simulink model "VDCHyd2022a"  (R2022a)
settings: Solver=daessc  StartTime=0.0  StopTime=simulationEndTime  FixedStep=0.001  RelTol=1e-2
values from neighbouring files (symbols this model uses):
  aux = thetaXrLB(i)    [initInertiaUpdate.m]
  Bc1_V = [0;0;0;0;0;0]    [InitializeSimulationParameters.m]
  Bc1_Vr = [0;0;0;0;0;0]    [InitializeSimulationParameters.m]
  D22Fr = [0;0;0;0;0;0]    [InitializeSimulationParameters.m]
  filtDF = init2ndOrderLowPassFilter(filtDF.cutOffFrequency,1,controller.dT)    [initializeLowPassFilters.m]
  filtDV = init2ndOrderLowPassFilter(filtDV.cutOffFrequency,1,controller.dT)    [initializeLowPassFilters.m]
  filtEnc = init2ndOrderLowPassFilter(filtEnc.cutOffFrequency,1,controller.dT)    [initializeLowPassFilters.m]
  filtPres = init2ndOrderLowPassFilter(filtPres.cutOffFrequency,1,controller.dT)    [initializeLowPassFilters.m]
  MODE = 1    [RUN_ME.m]
  s = tf('s')    [init2ndOrderLowPassFilter.m]
undefined symbols (not defined in the file or in its folder): B11_r_B11Tc1, B11_V, B11_Vr, B11Ftot_r, B12_r_B12Tc2, B12_Rot_Tc2, B12_U_Tc2, B12_V, B12_Vr, B12Ftot_r, B31_r_B31B41, B31_V, B31_Vr, B31FTot_r, B32_r_B32B42, B32_Rot_B42, B32_U_B42, B32_V, B32_Vr, B32FTot_r, B41_r_B41Tc1, B41_V, B41_Vr, B41FTot_r, B42_r_B42Tc2, B42_Rot_Tc2, B42_U_Tc2, B42_V, B42_Vr, B42FTot_r, B52_r_B52P32, B52_Rot_P32, B52_U_P32, B52_V, B52_Vr, B52Ftot_r, Bc1_r_Bc1B11, Bc1_r_Bc1B31, Bc1FTot_r, Bc2_r_Bc2B12, Bc2_r_Bc2B32, Bc2_Rot_B12, Bc2_Rot_B32, Bc2_U_B12, Bc2_U_B32, Bc2_V, Bc2_Vr, Bc2Tot_r, controller, cyl1, cyl2, cylT2, D22_V, D22_Vr, DiscIntNeverNeededParam, dq1, dq11, dq11r, dq12, dq12r ... (+119)
libraries: sm_lib x34, nesl_utility x15, simulink x11, dspinverses x1
(part 2 of 12)

== system VDCHyd2022a/sbHydraulicElements/sbHosesAndActuatorPS2 ==
  Qat2 : Inport
  Qbt2 : Inport  Port=2
  xt2 : Inport  Port=3
  dxt2 : Inport  Port=4
  sbChamberAPressure : Subsystem
  sbChamberBPressure : Subsystem
  sbLeakageFlow : Subsystem
  pat2 : Outport
  pbt2 : Outport  Port=2
  wires:
  sbChamberBPressure/1(pb) -> [pb]
  sbLeakageFlow/1(Ql) -> [Ql]
  sbChamberAPressure/1(pa) -> [pa]
  [dxp] -> sbChamberBPressure/4(dxp)
  [dxp] -> sbChamberAPressure/4(dxp)
  [xp] -> sbChamberAPressure/3(xp)
  [Qb] -> sbChamberBPressure/1(Qb)
  [xp] -> sbChamberBPressure/3(xp)
  [Ql] -> sbChamberBPressure/2(Ql)
  [Qa] -> sbChamberAPressure/1(Qa)
  [Ql] -> sbChamberAPressure/2(Ql)
  Qbt2/1 -> [Qb]  "Qbt2"
  Qat2/1 -> [Qa]  "Qat2"
  [pa] -> pat2/1  "pat2"
  [pb] -> pbt2/1  "pbt2"
  [pb] -> sbLeakageFlow/2(pb)
  [pa] -> sbLeakageFlow/1(pa)
  xt2/1 -> [xp]  "xt2"
  dxt2/1 -> [dxp]  "dxt2"

== system VDCHyd2022a/sbHydraulicElements/sbHosesAndActuatorRS1 ==
  Qa1 : Inport
  Qb1 : Inport  Port=2
  x1 : Inport  Port=3
  dx1 : Inport  Port=4
  sbChamberAPressure : Subsystem
  sbChamberBPressure : Subsystem
  sbLeakageFlow : Subsystem
  pa1 : Outport
  pb1 : Outport  Port=2
  wires:
  [dxp] -> sbChamberBPressure/4(dxp)
  [dxp] -> sbChamberAPressure/4(dxp)
  [xp] -> sbChamberAPressure/3(xp)
  [Qb] -> sbChamberBPressure/1(Qb)
  [xp] -> sbChamberBPressure/3(xp)
  [Ql] -> sbChamberBPressure/2(Ql)
  [Qa] -> sbChamberAPressure/1(Qa)
  [Ql] -> sbChamberAPressure/2(Ql)
  Qb1/1 -> [Qb]  "Qb1"
  Qa1/1 -> [Qa]  "Qa1"
  [pa] -> pa1/1  "pa1"
  [pb] -> pb1/1  "pb1"
  [pb] -> sbLeakageFlow/2(pb)
  [pa] -> sbLeakageFlow/1(pa)
  sbLeakageFlow/1(Ql) -> [Ql]
  x1/1 -> [xp]  "x1"
  dx1/1 -> [dxp]  "dx1"
  sbChamberBPressure/1(pb) -> [pb]
  sbChamberAPressure/1(pa) -> [pa]

== system VDCHyd2022a/sbHydraulicElements/sbHosesAndActuatorRS2 ==
  Qa2 : Inport
  Qb2 : Inport  Port=2
  x2 : Inport  Port=3
  dx2 : Inport  Port=4
  sbChamberAPressure : Subsystem
  sbChamberBPressure : Subsystem
  sbLeakageFlow : Subsystem
  pa2 : Outport
  pb2 : Outport  Port=2
  wires:
  dx2/1 -> [dxp]  "dx2"
  x2/1 -> [xp]  "x2"
  [pa] -> sbLeakageFlow/1(pa)
  [pb] -> sbLeakageFlow/2(pb)
  [pb] -> pb2/1  "pb2"
  [pa] -> pa2/1  "pa2"
  Qa2/1 -> [Qa]  "Qa2"
  Qb2/1 -> [Qb]  "Qb2"
  [Ql] -> sbChamberAPressure/2(Ql)
  [Qa] -> sbChamberAPressure/1(Qa)
  [Ql] -> sbChamberBPressure/2(Ql)
  [xp] -> sbChamberBPressure/3(xp)
  [Qb] -> sbChamberBPressure/1(Qb)
  [xp] -> sbChamberAPressure/3(xp)
  [dxp] -> sbChamberAPressure/4(dxp)
  [dxp] -> sbChamberBPressure/4(dxp)
  sbChamberAPressure/1(pa) -> [pa]  "pa"
  sbLeakageFlow/1(Ql) -> [Ql]  "Ql"
  sbChamberBPressure/1(pb) -> [pb]  "pb"

== system VDCHyd2022a/sbHydraulicElements/sbPistonForcePS2 ==
  note: f_{pt2} = A_{at2} p_{at2} - A_{bt2} p_{bt2}
  note: (79)
  pat2 : Inport
  pbt2 : Inport  Port=2
  Gain1 : Gain  Gain=cylT2.Aa
  Gain2 : Gain  Gain=cylT2.Ab
  Sum2 : Sum  Inputs=|+-
  fpt2 : Outport
  wires:
  Gain2/1 -> Sum2/2
  Sum2/1 -> fpt2/1  "fpt2"
  pat2/1 -> Gain1/1  "pat2"
  Gain1/1 -> Sum2/1
  pbt2/1 -> Gain2/1  "pbt2"

== system VDCHyd2022a/sbHydraulicElements/sbPistonForceRS1 ==
  note: f_{p1} = A_{a1} p_{a1} - A_{b1} p_{b1}
  note: (79)
  pa1 : Inport
  pb1 : Inport  Port=2
  Gain3 : Gain  Gain=cyl1.Aa
  Gain4 : Gain  Gain=cyl1.Ab
  Sum : Sum  Inputs=|+-
  fp1 : Outport
  wires:
  Gain3/1 -> Sum/1
  Gain4/1 -> Sum/2
  pb1/1 -> Gain4/1  "pb1"
  Sum/1 -> fp1/1  "fp1"
  pa1/1 -> Gain3/1  "pa1"

== system VDCHyd2022a/sbHydraulicElements/sbPistonForceRS2 ==
  note: (79)
  note: f_{p2} = A_{a2} p_{a2} - A_{b2} p_{b2}
  pa2 : Inport
  pb2 : Inport  Port=2
  Gain5 : Gain  Gain=cyl2.Aa
  Gain6 : Gain  Gain=cyl2.Ab
  Sum1 : Sum  Inputs=|+-
  fp2 : Outport
  wires:
  Gain6/1 -> Sum1/2
  Sum1/1 -> fp2/1  "fp2"
  Gain5/1 -> Sum1/1
  pb2/1 -> Gain6/1  "pb2"
  pa2/1 -> Gain5/1  "pa2"

== system VDCHyd2022a/sbHydraulicElements/sbPressureMeasurement ==
  pa1 : Inport
  pb1 : Inport  Port=2
  pa2 : Inport  Port=3
  pb2 : Inport  Port=4
  pat2 : Inport  Port=5
  pbt2 : Inport  Port=6
  pS : Inport  Port=7
  pR : Inport  Port=8
  Band-Limited White Noise{1..8} (8 alike) : simulink/Sources/Band-Limited White Noise  Cov=pres.measNoisePower  Ts=controller.dT  seed=[23341]
  Bus Creator1 : BusCreator  Inputs=pa1Measured,pb1Measured,pa2Measured,pb2Measured,pat2Measured,pbt2Measured,pSMeasured,pRMeasured
  Rate Transition : RateTransition  InitialCondition=initVals.pa10  OutPortSampleTime=controller.dT
  Rate Transition1 : RateTransition  InitialCondition=initVals.pb10  OutPortSampleTime=controller.dT
  Rate Transition2 : RateTransition  InitialCondition=initVals.pa20  OutPortSampleTime=controller.dT
  Rate Transition3 : RateTransition  InitialCondition=initVals.pb20  OutPortSampleTime=controller.dT
  Rate Transition4 : RateTransition  InitialCondition=initVals.pat20  OutPortSampleTime=controller.dT
  Rate Transition5 : RateTransition  InitialCondition=initVals.pbt20  OutPortSampleTime=controller.dT
  Rate Transition6 : RateTransition  InitialCondition=pres.supply  OutPortSampleTime=controller.dT
  Rate Transition7 : RateTransition  InitialCondition=pres.return  OutPortSampleTime=controller.dT
  Sum{3..10} (8 alike) : Sum  Inputs=|++
  pressuresMeasured : Outport
  wires:
  Sum4/1 -> Rate Transition1/1  "pb1Measured"
  Sum9/1 -> Rate Transition6/1  "pSMeasured"
  Sum7/1 -> Rate Transition4/1  "pat2Measured"
  Sum6/1 -> Rate Transition3/1  "pb2Measured"
  pS/1 -> Sum9/1
  Sum5/1 -> Rate Transition2/1  "pa2Measured"
  Band-Limited White Noise6/1 -> Sum3/2  "pa1MeasurementNoise"
  Band-Limited White Noise8/1 -> Sum10/2  "pRMeasurementNoise"
  pa2/1 -> Sum5/1
  Sum10/1 -> Rate Transition7/1  "pRMeasured"
  Rate Transition2/1 -> Bus Creator1/3  "pa2Measured"
  Sum8/1 -> Rate Transition5/1  "pbt2Measured"
  Rate Transition1/1 -> Bus Creator1/2  "pb1Measured"
  Rate Transition5/1 -> Bus Creator1/6  "pbt2Measured"
  pR/1 -> Sum10/1
  pat2/1 -> Sum7/1
  Rate Transition4/1 -> Bus Creator1/5  "pat2Measured"
  Rate Transition3/1 -> Bus Creator1/4  "pb2Measured"
  Rate Transition/1 -> Bus Creator1/1  "pa1Measured"
  Rate Transition7/1 -> Bus Creator1/8  "pRMeasured"
  Band-Limited White Noise2/1 -> Sum5/2  "pa2MeasurementNoise"
  Band-Limited White Noise5/1 -> Sum7/2  "pat2MeasurementNoise"
  Band-Limited White Noise3/1 -> Sum6/2  "pb2MeasurementNoise"
  Band-Limited White Noise4/1 -> Sum8/2  "pbt2MeasurementNoise"
  Sum3/1 -> Rate Transition/1  "pa1Measured"
  Band-Limited White Noise7/1 -> Sum9/2  "pSMeasurementNoise"
  Band-Limited White Noise1/1 -> Sum4/2  "pb1MeasurementNoise"
  pa1/1 -> Sum3/1
  Rate Transition6/1 -> Bus Creator1/7  "pSMeasured"
  Bus Creator1/1 -> pressuresMeasured/1  "pressuresMeasured"
  pb2/1 -> Sum6/1
  pbt2/1 -> Sum8/1
  pb1/1 -> Sum4/1

== system VDCHyd2022a/sbHydraulicElements/sbValve1SpoolDynamics ==
  note: NB! In the paper, u1v does not exist as a notion. High-bandwith valves are assumed to be used and u1v = u1. This is a fair assumption for valve like Bosch Rexroth NG6 size servo solenoid valve. Further tailoring valve dynamics per own needs could affect the flow and might require redoing control equations.
  u1 : Inport
  First Order Hold : FirstOrderHold  ErrorTolerance=inf
  rateLimiter : RateLimiter  RisingSlewLimit=valve1.riseSlewRate  FallingSlewLimit=valve1.fallSlewRate  SampleTimeMode=inherited
  saturation : Saturate  UpperLimit=valve1.uppLim  LowerLimit=valve1.lowLim
  spoolDynamics : TransferFcn  Numerator=[(valve1.nf)^2]  Denominator=[1 2*valve1.damp*(valve1.nf) (valve1.nf)^2]
  u1v : Outport
  wires:
  u1/1 -> First Order Hold/1  "u1"
  First Order Hold/1 -> saturation/1
  spoolDynamics/1 -> u1v/1  "u1v"
  rateLimiter/1 -> spoolDynamics/1
  saturation/1 -> rateLimiter/1

== system VDCHyd2022a/sbHydraulicElements/sbValve2SpoolDynamics ==
  note: NB! In the paper, u2v does not exist as a notion. High-bandwith valves are assumed to be used and u2v = u2. This is a fair assumption for valve like Bosch Rexroth NG6 size servo solenoid valve. Further tailoring valve dynamics per own needs could affect the flow and might require redoing control equations.
  u2 : Inport
  First Order Hold : FirstOrderHold  ErrorTolerance=inf
  rateLimiter : RateLimiter  RisingSlewLimit=valve2.riseSlewRate  FallingSlewLimit=valve2.fallSlewRate  SampleTimeMode=inherited
  saturation : Saturate  UpperLimit=valve2.uppLim  LowerLimit=valve2.lowLim
  spoolDynamics : TransferFcn  Numerator=[(valve2.nf)^2]  Denominator=[1 2*valve2.damp*(valve2.nf) (valve2.nf)^2]
  u2v : Outport
  wires:
  u2/1 -> First Order Hold/1  "u2"
  First Order Hold/1 -> saturation/1
  spoolDynamics/1 -> u2v/1  "u2v"
  saturation/1 -> rateLimiter/1
  rateLimiter/1 -> spoolDynamics/1

== system VDCHyd2022a/sbHydraulicElements/sbValveFlowsPS1 ==
  note: Q_{btj} = -c_{n2tj} \nu(p_{btj} - p_{r}) u_{tj} S(u_{tj}) - c_{p2tj} \nu (p_{S} - p_{btj}) u_{tj} S(-u_{tj})
  note: (83)
  note: (82)
  note: Q_{atj} = c_{p1tj} \nu(p_S - p_{atj}) u_{tj} S(u_{tj}) + c_{n1tj} \nu (p_{atj} - p_r) u_{tj} S(-u_{tj})
  pat2 : Inport
  pbt2 : Inport  Port=2
  ut2v : Inport  Port=3
  pS : Inport  Port=4
  pR : Inport  Port=5
  extensionValveFlows : MATLAB Function  TreatAsAtomicUnit=on
  Qat2 : Outport
  Qbt2 : Outport  Port=2
  wires:
  ut2v/1 -> extensionValveFlows/3(ut2v)  "ut2v"
  extensionValveFlows/1(Qat2) -> Qat2/1  "Qat2"
  pat2/1 -> extensionValveFlows/1(pat2)  "pat2"
  extensionValveFlows/2(Qbt2) -> Qbt2/1  "Qbt2"
  pR/1 -> extensionValveFlows/5(pR)  "pR"
  pS/1 -> extensionValveFlows/4(pS)  "pS"
  pbt2/1 -> extensionValveFlows/2(pbt2)  "pbt2"

== system VDCHyd2022a/sbHydraulicElements/sbValveFlowsRS1 ==
  note: (82)
  note: Q_{aj} = c_{p1j} \nu(p_S - p_{aj}) u_j S(u_j) + c_{n1j} \nu (p_{aj} - p_r) u_j S(-u_j)
  note: (83)
  note: Q_{bj} = -c_{n2j} \nu(p_{bj} - p_{r}) u_j S(u_j) - c_{p2j} \nu (p_{S} - p_{bj}) u_j S(-u_j)
  pa1 : Inport
  pb1 : Inport  Port=2
  u1v : Inport  Port=3
  pS : Inport  Port=4
  pR : Inport  Port=5
  liftValveFlows : MATLAB Function  TreatAsAtomicUnit=on
  Qa1 : Outport
  Qb1 : Outport  Port=2
  wires:
  u1v/1 -> liftValveFlows/3(u1v)  "u1v"
  pR/1 -> liftValveFlows/5(pR)  "pR"
  pb1/1 -> liftValveFlows/2(pb1)  "pb1"
  pS/1 -> liftValveFlows/4(pS)  "pS"
  liftValveFlows/1(Qa1) -> Qa1/1  "Qa1"
  liftValveFlows/2(Qb1) -> Qb1/1  "Qb1"
  pa1/1 -> liftValveFlows/1(pa1)  "pa1"

== system VDCHyd2022a/sbHydraulicElements/sbValveFlowsRS2 ==
  note: Q_{bj} = -c_{n2j} \nu(p_{bj} - p_{r}) u_j S(u_j) - c_{p2j} \nu (p_{S} - p_{bj}) u_j S(-u_j)
  note: (83)
  note: (82)
  note: Q_{aj} = c_{p1j} \nu(p_S - p_{aj}) u_j S(u_j) + c_{n1j} \nu (p_{aj} - p_r) u_j S(-u_j)
  pa2 : Inport
  pb2 : Inport  Port=2
  u2v : Inport  Port=3
  pS : Inport  Port=4
  pR : Inport  Port=5
  tiltValveFlows : MATLAB Function  TreatAsAtomicUnit=on
  Qa2 : Outport
  Qb2 : Outport  Port=2
  wires:
  u2v/1 -> tiltValveFlows/3(u2v)  "u2v"
  tiltValveFlows/1(Qa2) -> Qa2/1  "Qa2"
  pa2/1 -> tiltValveFlows/1(pa2)  "pa2"
  tiltValveFlows/2(Qb2) -> Qb2/1  "Qb2"
  pR/1 -> tiltValveFlows/5(pR)  "pR"
  pS/1 -> tiltValveFlows/4(pS)  "pS"
  pb2/1 -> tiltValveFlows/2(pb2)  "pb2"

== system VDCHyd2022a/sbHydraulicElements/sbValveT2SpoolDynamics ==
  note: NB! In the paper, ut2v does not exist as a notion. High-bandwith valves are assumed to be used and ut2v = ut2. This is a fair assumption for valve like Bosch Rexroth NG6 size servo solenoid valve. Further tailoring valve dynamics per own needs could affect the flow and might require redoing control equations.
  ut2 : Inport
  First Order Hold : FirstOrderHold  ErrorTolerance=inf
  rateLimiter : RateLimiter  RisingSlewLimit=valveT2.riseSlewRate  FallingSlewLimit=valveT2.fallSlewRate  SampleTimeMode=inherited
  saturation : Saturate  UpperLimit=valveT2.uppLim  LowerLimit=valveT2.lowLim
  spoolDynamics : TransferFcn  Numerator=[(valveT2.nf)^2]  Denominator=[1 2*valveT2.damp*(valveT2.nf) (valveT2.nf)^2]
  ut2v : Outport
  wires:
  ut2/1 -> First Order Hold/1  "ut2"
  First Order Hold/1 -> saturation/1
  spoolDynamics/1 -> ut2v/1  "ut2v"
  saturation/1 -> rateLimiter/1
  rateLimiter/1 -> spoolDynamics/1

== system VDCHyd2022a/sbHydraulicManipulatorSimscape/sbBase ==
  note: Defines world (W) frame.
  note: Resembles an ideal encoder.
  BaseR_To_W : sm_lib/Frames and Transforms/Rigid Transform  TranslationMethod=None  TranslationStandardOffset=0  TranslationLengthUnit=m  TranslationStandardAxis=+Z  TranslationCartesianOffset=[0 0 0]  TranslationROffset=0  TranslationROffsetUnits=m  TranslationZOffset=0  TranslationZOffsetUnits=m  TranslationThetaOffset=0  TranslationThetaOffsetUnits=deg  RotationMethod=StandardAxis  RotationAngleUnits=deg  RotationStandardAxis=+Y  RotationAngle=90  RotationArbitraryAxis=[0 0 1]  FollAlignAxisA=+X  BaseAlignAxisA=+Y  FollAlignAxisB=+Y  BaseAlignAxisB=+Z  RotationSequenceAxes=FollowerAxes  RotationSequence=XYX  RotationSequenceAngles=[0 0 0]  RotationSequenceAnglesUnits=deg  RotationMatrix=[1 0 0; 0 1 0; 0 0 1]
  BaseSolid : sm_lib/Body Elements/File Solid  ExtGeomFileName=01_BaseGP.STEP  UnitType=FromFile  ExtGeomFileUnits=m  StepReaderType=OCC  ExportConvexHullGeometry=off  InertiaType=Custom  Mass=307.29601379  MassUnits=kg  CenterOfMass=[0 -0.01488967 0.02139206]  CenterOfMassUnits=m  MomentsOfInertia=[29.78955950 5.25917100 29.30269608]  MomentsOfInertiaUnits=kg*m^2  ProductsOfInertia=[-3.89461427 -0.00003008 -0.00000910]  ProductsOfInertiaUnits=kg*m^2  BasedOnType=Density  Density=7300  DensityUnits=kg/m^3  DoExposeReferenceFrame=on  SerializedFrames=<Frames><Frame><Id>Frame1</Id><Value><Name>F2</Name><Origin><Source>GeometricFeature</Source><FeatureName>cylindrical surface 2</FeatureName></Origin><PrimaryAxis><DefinedDirection>+X</DefinedDirection><Source>ReferenceFrame</Source><SourceDirection>-Z</SourceDirection><FeatureName></FeatureName></PrimaryAxis><SecondaryAxis><DefinedDirection>+Y</DefinedDirection><Source>ReferenceFrame</Source><SourceDirection>+Y</SourceDirection><FeatureName></FeatureName></SecondaryAxis></Value></Frame><Frame><Id>Frame2</Id><Value><Name>F1</Name><Origin><Source>GeometricFeature</Source><FeatureName>cylindrical surface 1</FeatureName></Origin><PrimaryAxis><DefinedDirection>-X</DefinedDirection><Source>ReferenceFrame</Source><SourceDirection>+Z</SourceDirection><FeatureName></FeatureName></PrimaryAxis><SecondaryAxis><DefinedDirection>+Y</DefinedDirection><Source>ReferenceFrame</Source><SourceDirection>+Y</SourceDirection><FeatureName></FeatureName></SecondaryAxis></Value></Frame><Frame><Id>Frame3</Id><Value><Name>Bc1</Name><Origin><Source>GeometricFeature</Source><FeatureName>cylindrical surface 1</FeatureName></Origin><PrimaryAxis><DefinedDirection>+X</DefinedDirection><Source>GeometricFeature</Source><SourceDirection>+Z</SourceDirection><FeatureName>segment 135</FeatureName></PrimaryAxis><SecondaryAxis><DefinedDirection>+Y</DefinedDirection><Source>ReferenceFrame</Source><SourceDirection>+Z</SourceDirection><FeatureName></FeatureName></SecondaryAxis></Value></Frame></Frames>  GraphicType=FromGeometry  MarkerShape=Sphere  MarkerSize=10  GraphicVisPropType=SimpleVisualProperties  GraphicDiffuseColor=[134 134 71]/255  GraphicSpecularColor=[0.5 0.5 0.5 1.0]  GraphicAmbientColor=[0.15 0.15 0.15 1.0]  GraphicEmissiveColor=[0.0 0.0 0.0 1.0]  GraphicShininess=75  GraphicOpacity=1.0
  PS-Simulink Converter : nesl_utility/PS-Simulink Converter  PhysicalDomain=network_engine_domain  SubClassName=ps_output  LeftPortType=input  RightPortType=output  PseudoPeriodic=off  Frequencies=[]  VectorFormat=inherit  Unit=inherit  AffineConversion=off
      settings: SourceProductBaseCode=SS,PW,VE
  theta1Rotation : sm_lib/Joints/Revolute Joint  JointMode=Normal  SenseConstraintForce=off  SenseConstraintForceX=off  SenseConstraintForceY=off  SenseConstraintForceZ=off  SenseConstraintTorque=off  SenseConstraintTorqueX=off  SenseConstraintTorqueY=off  SenseConstraintTorqueZ=off  SenseTotalForce=off  SenseTotalForceX=off  SenseTotalForceY=off  SenseTotalForceZ=off  SenseTotalTorque=off  SenseTotalTorqueX=off  SenseTotalTorqueY=off  SenseTotalTorqueZ=off  CompositeWrenchDir=FollowerOnBase  CompositeWrenchFrame=BaseFrame  EquilibriumPosition=0  EquilibriumPositionUnits=rad  SpringStiffness=0  SpringStiffnessUnits=N*m/rad  DampingCoefficient=revJoint1.damp  DampingCoefficientUnits=N*m/(rad/s)  TorqueActuationMode=NoTorque  MotionActuationMode=ComputedMotion  SensePosition=on  SenseVelocity=off  SenseAcceleration=off  SenseTorqueForce=off  SenseLowerLimitTorqueForce=off  SenseUpperLimitTorqueForce=off  LowerLimitSpecify=off  LowerLimitBound=-90  LowerLimitBoundUnits=deg  LowerLimitStiffness=1e4  LowerLimitStiffnessUnits=N*m/deg  LowerLimitDamping=10  LowerLimitDampingUnits=N*m/(deg/s)  LowerLimitTransitionRegionWidth=0.1  LowerLimitTransitionRegionWidthUnits=deg  UpperLimitSpecify=off  UpperLimitBound=90  UpperLimitBoundUnits=deg  UpperLimitStiffness=1e4  UpperLimitStiffnessUnits=N*m/deg  UpperLimitDamping=10  UpperLimitDampingUnits=N*m/(deg/s)  UpperLimitTransitionRegionWidth=0.1  UpperLimitTransitionRegionWidthUnits=deg  PositionTargetSpecify=on  PositionTargetPriority=High  PositionTargetValue=initVals.theta10  PositionTargetValueUnits=rad  VelocityTargetSpecify=on  VelocityTargetPriority=High  VelocityTargetValue=0  VelocityTargetValueUnits=rad/s
  W : PMIOPort  Side=Left
  Bc1 : PMIOPort  Port=2  Side=Left
  F1 : PMIOPort  Port=3  Side=Right
  F2_rot : PMIOPort  Port=4  Side=Right
  theta1 : Outport
  wires:
  PS-Simulink Converter/1 -> theta1/1
  connections:
  BaseR_To_W/LConn1 -- BaseSolid/RConn1
  W/RConn1 -- BaseR_To_W/RConn1
  theta1Rotation/LConn1 -- BaseSolid/LConn1
  F2_rot/RConn1 -- theta1Rotation/RConn1
  F1/RConn1 -- BaseSolid/LConn2
  Bc1/RConn1 -- BaseSolid/RConn2
  PS-Simulink Converter/LConn1 -- theta1Rotation/RConn2

== system VDCHyd2022a/sbHydraulicManipulatorSimscape/sbEndMassObject ==
  EndObjectMass : sm_lib/Body Elements/File Solid  ExtGeomFileName=10_ObjectGP.STEP  UnitType=FromFile  ExtGeomFileUnits=m  StepReaderType=OCC  ExportConvexHullGeometry=off  InertiaType=Custom  Mass=570.18877059  MassUnits=kg  CenterOfMass=[2.16142487 0.01347152 0.06601658]  CenterOfMassUnits=m  MomentsOfInertia=[46.81220713 72.19317437 67.11012925]  MomentsOfInertiaUnits=kg*m^2  ProductsOfInertia=[0.04641137 0.08825278 0.37588204]  ProductsOfInertiaUnits=kg*m^2  BasedOnType=Density  Density=7850  DensityUnits=kg/m^3  DoExposeReferenceFrame=off  SerializedFrames=<Frames><Frame><Id>Frame1</Id><Value><Name>P32p</Name><Origin><Source>GeometricFeature</Source><FeatureName>circular curve 7</FeatureName></Origin><PrimaryAxis><DefinedDirection>+Y</DefinedDirection><Source>GeometricFeature</Source><SourceDirection>+Z</SourceDirection><FeatureName>segment 159</FeatureName></PrimaryAxis><SecondaryAxis><DefinedDirection>+X</DefinedDirection><Source>ReferenceFrame</Source><SourceDirection>+X</SourceDirection><FeatureName></FeatureName></SecondaryAxis></Value></Frame><Frame><Id>Frame2</Id><Value><Name>D22</Name><Origin><Source>GeometricFeature</Source><FeatureName>planar surface 154</FeatureName></Origin><PrimaryAxis><DefinedDirection>+Z</DefinedDirection><Source>ReferenceFrame</Source><SourceDirection>+Z</SourceDirection><FeatureName></FeatureName></PrimaryAxis><SecondaryAxis><DefinedDirection>+X</DefinedDirection><Source>ReferenceFrame</Source><SourceDirection>+X</SourceDirection><FeatureName></FeatureName></SecondaryAxis></Value></Frame></Frames>  GraphicType=FromGeometry  MarkerShape=Sphere  MarkerSize=10  GraphicVisPropType=SimpleVisualProperties  GraphicDiffuseColor=[255 9 134]/255  GraphicSpecularColor=[0.5 0.5 0.5 1.0]  GraphicAmbientColor=[0.15 0.15 0.15 1.0]  GraphicEmissiveColor=[0.0 0.0 0.0 1.0]  GraphicShininess=75  GraphicOpacity=1.0
  P32p_to_P32 : sm_lib/Frames and Transforms/Rigid Transform  TranslationMethod=StandardAxis  TranslationStandardOffset=17  TranslationLengthUnit=mm  TranslationStandardAxis=+Z  TranslationCartesianOffset=[0 0 0]  TranslationROffset=0  TranslationROffsetUnits=m  TranslationZOffset=0  TranslationZOffsetUnits=m  TranslationThetaOffset=0  TranslationThetaOffsetUnits=deg  RotationMethod=None  RotationAngleUnits=deg  RotationStandardAxis=+Y  RotationAngle=-90  RotationArbitraryAxis=[0 0 1]  FollAlignAxisA=+X  BaseAlignAxisA=+Y  FollAlignAxisB=+Y  BaseAlignAxisB=+Z  RotationSequenceAxes=FollowerAxes  RotationSequence=XYX  RotationSequenceAngles=[0 0 0]  RotationSequenceAnglesUnits=deg  RotationMatrix=[1 0 0; 0 1 0; 0 0 1]
  P32 : PMIOPort  Side=Left
  D22 : PMIOPort  Port=2  Side=Left
  connections:
  EndObjectMass/LConn1 -- P32p_to_P32/LConn1
  P32p_to_P32/RConn1 -- P32/RConn1
  D22/RConn1 -- EndObjectMass/RConn1

== system VDCHyd2022a/sbHydraulicManipulatorSimscape/sbLiftCylinderAndLiftPiston ==
  note: Friction force...
  fp1 : Inport
  B31p_to_B31pAux : sm_lib/Frames and Transforms/Rigid Transform  TranslationMethod=None  TranslationStandardOffset=0  TranslationLengthUnit=m  TranslationStandardAxis=+Z  TranslationCartesianOffset=[0 0 0]  TranslationROffset=0  TranslationROffsetUnits=m  TranslationZOffset=0  TranslationZOffsetUnits=m  TranslationThetaOffset=0  TranslationThetaOffsetUnits=deg  RotationMethod=StandardAxis  RotationAngleUnits=deg  RotationStandardAxis=+Y  RotationAngle=90  RotationArbitraryAxis=[0 0 1]  FollAlignAxisA=+X  BaseAlignAxisA=+Y  FollAlignAxisB=+Y  BaseAlignAxisB=+Z  RotationSequenceAxes=FollowerAxes  RotationSequence=XYX  RotationSequenceAngles=[0 0 0]  RotationSequenceAnglesUnits=deg  RotationMatrix=[1 0 0; 0 1 0; 0 0 1]
  B41Aux_to_B41 : sm_lib/Frames and Transforms/Rigid Transform  TranslationMethod=None  TranslationStandardOffset=0  TranslationLengthUnit=m  TranslationStandardAxis=+Z  TranslationCartesianOffset=[0 0 0]  TranslationROffset=0  TranslationROffsetUnits=m  TranslationZOffset=0  TranslationZOffsetUnits=m  TranslationThetaOffset=0  TranslationThetaOffsetUnits=deg  RotationMethod=StandardAxis  RotationAngleUnits=deg  RotationStandardAxis=+Y  RotationAngle=-90  RotationArbitraryAxis=[0 0 1]  FollAlignAxisA=+X  BaseAlignAxisA=+Y  FollAlignAxisB=+Y  BaseAlignAxisB=+Z  RotationSequenceAxes=FollowerAxes  RotationSequence=XYX  RotationSequenceAngles=[0 0 0]  RotationSequenceAnglesUnits=deg  RotationMatrix=[1 0 0; 0 1 0; 0 0 1]
  Constant : Constant  Value=settings.actuatorFrictionON
  Constant1 : Constant  Value=0
  LiftCylinderSolid : sm_lib/Body Elements/File Solid  ExtGeomFileName=03_LiftCylGP.STEP  UnitType=FromFile  ExtGeomFileUnits=m  StepReaderType=OCC  ExportConvexHullGeometry=off  InertiaType=Custom  Mass=17.36281648  MassUnits=kg  CenterOfMass=[0 0.31781210 0]  CenterOfMassUnits=m  MomentsOfInertia=[0.90735702 0.03150902 0.90763033]  MomentsOfInertiaUnits=kg*m^2  ProductsOfInertia=[0 0 0]  ProductsOfInertiaUnits=kg*m^2  BasedOnType=Density  Density=7300  DensityUnits=kg/m^3  DoExposeReferenceFrame=off  SerializedFrames=<Frames><Frame><Id>Frame1</Id><Value><Name>B31</Name><Origin><Source>GeometricFeature</Source><FeatureName>cylindrical surface 11</FeatureName></Origin><PrimaryAxis><DefinedDirection>+X</DefinedDirection><Source>ReferenceFrame</Source><SourceDirection>+Y</SourceDirection><FeatureName></FeatureName></PrimaryAxis><SecondaryAxis><DefinedDirection>+Y</DefinedDirection><Source>ReferenceFrame</Source><SourceDirection>-X</SourceDirection><FeatureName></FeatureName></SecondaryAxis></Value></Frame><Frame><Id>Frame2</Id><Value><Name>B31p</Name><Origin><Source>GeometricFeature</Source><FeatureName>planar surface 4</FeatureName></Origin><PrimaryAxis><DefinedDirection>+X</DefinedDirection><Source>ReferenceFrame</Source><SourceDirection>+Y</SourceDirection><FeatureName></FeatureName></PrimaryAxis><SecondaryAxis><DefinedDirection>+Y</DefinedDirection><Source>ReferenceFrame</Source><SourceDirection>-X</SourceDirection><FeatureName></FeatureName></SecondaryAxis></Value></Frame></Frames>  GraphicType=FromGeometry  MarkerShape=Sphere  MarkerSize=10  GraphicVisPropType=SimpleVisualProperties  GraphicDiffuseColor=[1 1 119]/255  GraphicSpecularColor=[0.5 0.5 0.5 1.0]  GraphicAmbientColor=[0.15 0.15 0.15 1.0]  GraphicEmissiveColor=[0.0 0.0 0.0 1.0]  GraphicShininess=75  GraphicOpacity=1.0
  LiftPistonSolid : sm_lib/Body Elements/File Solid  ExtGeomFileName=04_LiftPistGP.STEP  UnitType=FromFile  ExtGeomFileUnits=m  StepReaderType=OCC  ExportConvexHullGeometry=off  InertiaType=Custom  Mass=10.34519231  MassUnits=kg  CenterOfMass=[0 0.32981882 0]  CenterOfMassUnits=m  MomentsOfInertia=[0.55759812 0.00370720 0.55785997]  MomentsOfInertiaUnits=kg*m^2  ProductsOfInertia=[0 0 0]  ProductsOfInertiaUnits=kg*m^2  BasedOnType=Density  Density=7800  DensityUnits=kg/m^3  DoExposeReferenceFrame=off  SerializedFrames=<Frames><Frame><Id>Frame2</Id><Value><Name>B41</Name><Origin><Source>GeometricFeature</Source><FeatureName>planar surface 2</FeatureName></Origin><PrimaryAxis><DefinedDirection>+X</DefinedDirection><Source>ReferenceFrame</Source><SourceDirection>+Y</SourceDirection><FeatureName></FeatureName></PrimaryAxis><SecondaryAxis><DefinedDirection>+Y</DefinedDirection><Source>ReferenceFrame</Source><SourceDirection>-X</SourceDirection><FeatureName></FeatureName></SecondaryAxis></Value></Frame><Frame><Id>Frame3</Id><Value><Name>P11</Name><Origin><Source>GeometricFeature</Source><FeatureName>cylindrical surface 8</FeatureName></Origin><PrimaryAxis><DefinedDirection>+X</DefinedDirection><Source>ReferenceFrame</Source><SourceDirection>+Y</SourceDirection><FeatureName></FeatureName></PrimaryAxis><SecondaryAxis><DefinedDirection>+Y</DefinedDirection><Source>ReferenceFrame</Source><SourceDirection>-X</SourceDirection><FeatureName></FeatureName></SecondaryAxis></Value></Frame></Frames>  GraphicType=FromGeometry  MarkerShape=Sphere  MarkerSize=10  GraphicVisPropType=SimpleVisualProperties  GraphicDiffuseColor=[9 232 232]/255  GraphicSpecularColor=[0.5 0.5 0.5 1.0]  GraphicAmbientColor=[0.15 0.15 0.15 1.0]  GraphicEmissiveColor=[0.0 0.0 0.0 1.0]  GraphicShininess=75  GraphicOpacity=1.0
  PS-Sim1 : nesl_utility/PS-Simulink Converter  PhysicalDomain=network_engine_domain  SubClassName=ps_output  LeftPortType=input  RightPortType=output  PseudoPeriodic=off  Frequencies=[]  VectorFormat=1-D array  Unit=inherit  AffineConversion=off
      settings: SourceProductBaseCode=SS,PW,VE
  PS-Sim2 : nesl_utility/PS-Simulink Converter  PhysicalDomain=network_engine_domain  SubClassName=ps_output  LeftPortType=input  RightPortType=output  PseudoPeriodic=off  Frequencies=[]  VectorFormat=1-D array  Unit=inherit  AffineConversion=off
      settings: SourceProductBaseCode=SS,PW,VE
  Simulink-PS Converter : nesl_utility/Simulink-PS Converter  PhysicalDomain=network_engine_domain  SubClassName=ps_input  LeftPortType=input  RightPortType=output  PseudoPeriodic=off  Frequencies=[]  NoiseDistribution=none  NoiseParameters=[]  Unit=1  AffineConversion=off  FilteringAndDerivatives=provide  SimscapeFilterOrder=1  InputFilterTimeConstant=0.001  UdotUserProvided=0
      settings: SourceProductBaseCode=SS,PW,VE
  Sum : Sum  Inputs=|+-
  Switch : Switch  Criteria=u2 > Threshold  SaturateOnIntegerOverflow=off  InputSameDT=off
  q11Rotation : sm_lib/Joints/Revolute Joint  JointMode=Normal  SenseConstraintForce=off  SenseConstraintForceX=off  SenseConstraintForceY=off  SenseConstraintForceZ=off  SenseConstraintTorque=off  SenseConstraintTorqueX=off  SenseConstraintTorqueY=off  SenseConstraintTorqueZ=off  SenseTotalForce=off  SenseTotalForceX=off  SenseTotalForceY=off  SenseTotalForceZ=off  SenseTotalTorque=off  SenseTotalTorqueX=off  SenseTotalTorqueY=off  SenseTotalTorqueZ=off  CompositeWrenchDir=FollowerOnBase  CompositeWrenchFrame=BaseFrame  EquilibriumPosition=0  EquilibriumPositionUnits=rad  SpringStiffness=0  SpringStiffnessUnits=N*m/rad  DampingCoefficient=revJoint1.damp  DampingCoefficientUnits=N*m/(rad/s)  TorqueActuationMode=NoTorque  MotionActuationMode=ComputedMotion  SensePosition=off  SenseVelocity=off  SenseAcceleration=off  SenseTorqueForce=off  SenseLowerLimitTorqueForce=off  SenseUpperLimitTorqueForce=off  LowerLimitSpecify=off  LowerLimitBound=-90  LowerLimitBoundUnits=deg  LowerLimitStiffness=1e4  LowerLimitStiffnessUnits=N*m/deg  LowerLimitDamping=10  LowerLimitDampingUnits=N*m/(deg/s)  LowerLimitTransitionRegionWidth=0.1  LowerLimitTransitionRegionWidthUnits=deg  UpperLimitSpecify=off  UpperLimitBound=90  UpperLimitBoundUnits=deg  UpperLimitStiffness=1e4  UpperLimitStiffnessUnits=N*m/deg  UpperLimitDamping=10  UpperLimitDampingUnits=N*m/(deg/s)  UpperLimitTransitionRegionWidth=0.1  UpperLimitTransitionRegionWidthUnits=deg  PositionTargetSpecify=off  PositionTargetPriority=High  PositionTargetValue=0  PositionTargetValueUnits=deg  VelocityTargetSpecify=off  VelocityTargetPriority=High  VelocityTargetValue=0  VelocityTargetValueUnits=deg/s
  q12Rotation : sm_lib/Joints/Revolute Joint  JointMode=Normal  SenseConstraintForce=off  SenseConstraintForceX=off  SenseConstraintForceY=off  SenseConstraintForceZ=off  SenseConstraintTorque=off  SenseConstraintTorqueX=off  SenseConstraintTorqueY=off  SenseConstraintTorqueZ=off  SenseTotalForce=off  SenseTotalForceX=off  SenseTotalForceY=off  SenseTotalForceZ=off  SenseTotalTorque=off  SenseTotalTorqueX=off  SenseTotalTorqueY=off  SenseTotalTorqueZ=off  CompositeWrenchDir=FollowerOnBase  CompositeWrenchFrame=BaseFrame  EquilibriumPosition=0  EquilibriumPositionUnits=rad  SpringStiffness=0  SpringStiffnessUnits=N*m/rad  DampingCoefficient=revJoint1.damp  DampingCoefficientUnits=N*m/(rad/s)  TorqueActuationMode=NoTorque  MotionActuationMode=ComputedMotion  SensePosition=off  SenseVelocity=off  SenseAcceleration=off  SenseTorqueForce=off  SenseLowerLimitTorqueForce=off  SenseUpperLimitTorqueForce=off  LowerLimitSpecify=off  LowerLimitBound=-90  LowerLimitBoundUnits=deg  LowerLimitStiffness=1e4  LowerLimitStiffnessUnits=N*m/deg  LowerLimitDamping=10  LowerLimitDampingUnits=N*m/(deg/s)  LowerLimitTransitionRegionWidth=0.1  LowerLimitTransitionRegionWidthUnits=deg  UpperLimitSpecify=off  UpperLimitBound=90  UpperLimitBoundUnits=deg  UpperLimitStiffness=1e4  UpperLimitStiffnessUnits=N*m/deg  UpperLimitDamping=10  UpperLimitDampingUnits=N*m/(deg/s)  UpperLimitTransitionRegionWidth=0.1  UpperLimitTransitionRegionWidthUnits=deg  PositionTargetSpecify=off  PositionTargetPriority=High  PositionTargetValue=0  PositionTargetValueUnits=deg  VelocityTargetSpecify=off  VelocityTargetPriority=High  VelocityTargetValue=0  VelocityTargetValueUnits=deg/s
  sbFrictionForceRS1 : Subsystem
  x1-translation : sm_lib/Joints/Prismatic Joint  JointMode=Normal  SenseConstraintForce=off  SenseConstraintForceX=off  SenseConstraintForceY=off  SenseConstraintForceZ=off  SenseConstraintTorque=off  SenseConstraintTorqueX=off  SenseConstraintTorqueY=off  SenseConstraintTorqueZ=off  SenseTotalForce=off  SenseTotalForceX=off  SenseTotalForceY=off  SenseTotalForceZ=off  SenseTotalTorque=off  SenseTotalTorqueX=off  SenseTotalTorqueY=off  SenseTotalTorqueZ=off  CompositeWrenchDir=FollowerOnBase  CompositeWrenchFrame=FollowerFrame  EquilibriumPosition=0  EquilibriumPositionUnits=m  SpringStiffness=0  SpringStiffnessUnits=N/m  DampingCoefficient=0  DampingCoefficientUnits=N/(m/s)  TorqueActuationMode=InputTorque  MotionActuationMode=ComputedMotion  SensePosition=on  SenseVelocity=on  SenseAcceleration=off  SenseTorqueForce=off  SenseLowerLimitTorqueForce=off  SenseUpperLimitTorqueForce=off  LowerLimitSpecify=on  LowerLimitBound=0  LowerLimitBoundUnits=m  LowerLimitStiffness=1e6  LowerLimitStiffnessUnits=N/m  LowerLimitDamping=1e3  LowerLimitDampingUnits=N/(m/s)  LowerLimitTransitionRegionWidth=1e-4  LowerLimitTransitionRegionWidthUnits=m  UpperLimitSpecify=on  UpperLimitBound=cyl1.sp  UpperLimitBoundUnits=m  UpperLimitStiffness=1e6  UpperLimitStiffnessUnits=N/m  UpperLimitDamping=1e3  UpperLimitDampingUnits=N/(m/s)  UpperLimitTransitionRegionWidth=1e-4  UpperLimitTransitionRegionWidthUnits=m  PositionTargetSpecify=on  PositionTargetPriority=Low  PositionTargetValue=0.4  PositionTargetValueUnits=m  VelocityTargetSpecify=on  VelocityTargetPriority=High  VelocityTargetValue=0  VelocityTargetValueUnits=m/s
  B31 : PMIOPort  Side=Left
  B41 : PMIOPort  Port=2  Side=Left
  F1 : PMIOPort  Port=3  Side=Right
  F3 : PMIOPort  Port=4  Side=Right
  x1 : Outport
  dx1 : Outport  Port=2
  wires:
  PS-Sim1/1 -> x1/1
  fp1/1 -> sbFrictionForceRS1/2(fp1), Sum/1
  Sum/1 -> Simulink-PS Converter/1
  Switch/1 -> Sum/2
  PS-Sim2/1 -> sbFrictionForceRS1/1(dx1), dx1/1
  Constant1/1 -> Switch/3
  sbFrictionForceRS1/1(ff1) -> Switch/1
  Constant/1 -> Switch/2
  connections:
  B31p_to_B31pAux/LConn1 -- LiftCylinderSolid/RConn1
  x1-translation/RConn1 -- B41Aux_to_B41/LConn1
  q11Rotation/RConn1 -- B31/RConn1 -- LiftCylinderSolid/LConn1
  LiftPistonSolid/LConn1 -- B41/RConn1 -- B41Aux_to_B41/RConn1
  B31p_to_B31pAux/RConn1 -- x1-translation/LConn1
  q11Rotation/LConn1 -- F1/RConn1
  q12Rotation/LConn1 -- LiftPistonSolid/RConn1
  q12Rotation/RConn1 -- F3/RConn1
  PS-Sim1/LConn1 -- x1-translation/RConn2
  Simulink-PS Converter/RConn1 -- x1-translation/LConn2
  x1-translation/RConn3 -- PS-Sim2/LConn1

== system VDCHyd2022a/sbHydraulicManipulatorSimscape/sbLiftLink ==
  note: Resembles an ideal encoder.
  LiftLinkSolid : sm_lib/Body Elements/File Solid  ExtGeomFileName=02_LiftLinkGP.STEP  UnitType=FromFile  ExtGeomFileUnits=m  StepReaderType=OCC  ExportConvexHullGeometry=off  InertiaType=Custom  Mass=80.11363010  MassUnits=kg  CenterOfMass=[0 -0.04248930 0.76135480]  CenterOfMassUnits=m  MomentsOfInertia=[16.37344274 16.11821222 0.72023904]  MomentsOfInertiaUnits=kg*m^2  ProductsOfInertia=[-0.55980815 0 0]  ProductsOfInertiaUnits=kg*m^2  BasedOnType=Mass  Density=7300  DensityUnits=kg/m^3  DoExposeReferenceFrame=off  SerializedFrames=<Frames><Frame><Id>Frame1</Id><Value><Name>F5</Name><Origin><Source>GeometricFeature</Source><FeatureName>cylindrical surface 18</FeatureName></Origin><PrimaryAxis><DefinedDirection>+X</DefinedDirection><Source>ReferenceFrame</Source><SourceDirection>+Z</SourceDirection><FeatureName></FeatureName></PrimaryAxis><SecondaryAxis><DefinedDirection>+Y</DefinedDirection><Source>ReferenceFrame</Source><SourceDirection>+Y</SourceDirection><FeatureName></FeatureName></SecondaryAxis></Value></Frame><Frame><Id>Frame2</Id><Value><Name>F2rot</Name><Origin><Source>GeometricFeature</Source><FeatureName>cylindrical surface 7</FeatureName></Origin><PrimaryAxis><DefinedDirection>+X</DefinedDirection><Source>ReferenceFrame</Source><SourceDirection>+Z</SourceDirection><FeatureName></FeatureName></PrimaryAxis><SecondaryAxis><DefinedDirection>+Y</DefinedDirection><Source>ReferenceFrame</Source><SourceDirection>+Y</SourceDirection><FeatureName></FeatureName></SecondaryAxis></Value></Frame><Frame><Id>Frame3</Id><Value><Name>F3</Name><Origin><Source>GeometricFeature</Source><FeatureName>cylindrical surface 8</FeatureName></Origin><PrimaryAxis><DefinedDirection>+X</DefinedDirection><Source>ReferenceFrame</Source><SourceDirection>+Z</SourceDirection><FeatureName></FeatureName></PrimaryAxis><SecondaryAxis><DefinedDirection>+Y</DefinedDirection><Source>ReferenceFrame</Source><SourceDirection>+Y</SourceDirection><FeatureName></FeatureName></SecondaryAxis></Value></Frame><Frame><Id>Frame4</Id><Value><Name>F4</Name><Origin><Source>GeometricFeature</Source><FeatureName>cylindrical surface 9</FeatureName></Origin><PrimaryAxis><DefinedDirection>+X</DefinedDirection><Source>ReferenceFrame</Source><SourceDirection>+Z</SourceDirection><FeatureName></FeatureName></PrimaryAxis><SecondaryAxis><DefinedDirection>+Y</DefinedDirection><Source>ReferenceFrame</Source><SourceDirection>+Y</SourceDirection><FeatureName></FeatureName></SecondaryAxis></Value></Frame><Frame><Id>Frame5</Id><Value><Name>B11</Name><Origin><Source>GeometricFeature</Source><FeatureName>cylindrical surface 7</FeatureName></Origin><PrimaryAxis><DefinedDirection>+X</DefinedDirection><Source>GeometricFeature</Source><SourceDirection>+Z</SourceDirection><FeatureName>segment 149</FeatureName></PrimaryAxis><SecondaryAxis><DefinedDirection>+Y</DefinedDirection><Source>ReferenceFrame</Source><SourceDirection>+Y</SourceDirection><FeatureName></FeatureName></SecondaryAxis></Value></Frame><Frame><Id>Frame6</Id><Value><Name>Bc2</Name><Origin><Source>GeometricFeature</Source><FeatureName>cylindrical surface 9</FeatureName></Origin><PrimaryAxis><DefinedDirection>+X</DefinedDirection><Source>GeometricFeature</Source><SourceDirection>+Z</SourceDirection><FeatureName>segment 153</FeatureName></PrimaryAxis><SecondaryAxis><DefinedDirection>+Y</DefinedDirection><Source>ReferenceFrame</Source><SourceDirection>+Y</SourceDirection><FeatureName></FeatureName></SecondaryAxis></Value></Frame><Frame><Id>Frame7</Id><Value><Name>Tc1</Name><Origin><Source>GeometricFeature</Source><FeatureName>cylindrical surface 8</FeatureName></Origin><PrimaryAxis><DefinedDirection>+X</DefinedDirection><Source>GeometricFeature</Source><SourceDirection>+Z</SourceDirection><FeatureName>segment 149</FeatureName></PrimaryAxis><SecondaryAxis><DefinedDirection>+Y</DefinedDirection><Source>ReferenceFrame</Source><SourceDirection>+Y</SourceDirection><FeatureName></FeatureName></SecondaryAxis></Value></Frame></Frames>  GraphicType=FromGeometry  MarkerShape=Sphere  MarkerSize=10  GraphicVisPropType=SimpleVisualProperties  GraphicDiffuseColor=[255 192 138]/255  GraphicSpecularColor=[0.5 0.5 0.5 1.0]  GraphicAmbientColor=[0.15 0.15 0.15 1.0]  GraphicEmissiveColor=[0.0 0.0 0.0 1.0]  GraphicShininess=75  GraphicOpacity=1.0
  PS-Simulink Converter : nesl_utility/PS-Simulink Converter  PhysicalDomain=network_engine_domain  SubClassName=ps_output  LeftPortType=input  RightPortType=output  PseudoPeriodic=off  Frequencies=[]  VectorFormat=inherit  Unit=inherit  AffineConversion=off
      settings: SourceProductBaseCode=SS,PW,VE
  theta2Rotation : sm_lib/Joints/Revolute Joint  JointMode=Normal  SenseConstraintForce=off  SenseConstraintForceX=off  SenseConstraintForceY=off  SenseConstraintForceZ=off  SenseConstraintTorque=off  SenseConstraintTorqueX=off  SenseConstraintTorqueY=off  SenseConstraintTorqueZ=off  SenseTotalForce=off  SenseTotalForceX=off  SenseTotalForceY=off  SenseTotalForceZ=off  SenseTotalTorque=off  SenseTotalTorqueX=off  SenseTotalTorqueY=off  SenseTotalTorqueZ=off  CompositeWrenchDir=FollowerOnBase  CompositeWrenchFrame=BaseFrame  EquilibriumPosition=0  EquilibriumPositionUnits=deg  SpringStiffness=0  SpringStiffnessUnits=N*m/deg  DampingCoefficient=revJoint2.damp  DampingCoefficientUnits=N*m/(deg/s)  TorqueActuationMode=NoTorque  MotionActuationMode=ComputedMotion  SensePosition=on  SenseVelocity=off  SenseAcceleration=off  SenseTorqueForce=off  SenseLowerLimitTorqueForce=off  SenseUpperLimitTorqueForce=off  LowerLimitSpecify=off  LowerLimitBound=-90  LowerLimitBoundUnits=deg  LowerLimitStiffness=1e4  LowerLimitStiffnessUnits=N*m/deg  LowerLimitDamping=10  LowerLimitDampingUnits=N*m/(deg/s)  LowerLimitTransitionRegionWidth=0.1  LowerLimitTransitionRegionWidthUnits=deg  UpperLimitSpecify=off  UpperLimitBound=90  UpperLimitBoundUnits=deg  UpperLimitStiffness=1e4  UpperLimitStiffnessUnits=N*m/deg  UpperLimitDamping=10  UpperLimitDampingUnits=N*m/(deg/s)  UpperLimitTransitionRegionWidth=0.1  UpperLimitTransitionRegionWidthUnits=deg  PositionTargetSpecify=on  PositionTargetPriority=High  PositionTargetValue=initVals.theta20  PositionTargetValueUnits=rad  VelocityTargetSpecify=on  VelocityTargetPriority=High  VelocityTargetValue=0  VelocityTargetValueUnits=rad/s
  F4 : PMIOPort  Side=Left
  F5_rot : PMIOPort  Port=2  Side=Left
  F3 : PMIOPort  Port=3  Side=Left
  F2_rot : PMIOPort  Port=4  Side=Right
  Bc2 : PMIOPort  Port=5  Side=Right
  B11 : PMIOPort  Port=6  Side=Right
  Tc1 : PMIOPort  Port=7  Side=Right
  theta2 : Outport
  wires:
  PS-Simulink Converter/1 -> theta2/1
  connections:
  theta2Rotation/RConn1 -- F5_rot/RConn1
  F2_rot/RConn1 -- LiftLinkSolid/RConn1
  LiftLinkSolid/LConn2 -- F3/RConn1
  F4/RConn1 -- LiftLinkSolid/RConn2
  LiftLinkSolid/LConn1 -- theta2Rotation/LConn1
  LiftLinkSolid/LConn3 -- B11/RConn1
  LiftLinkSolid/LConn4 -- Tc1/RConn1
  Bc2/RConn1 -- LiftLinkSolid/RConn3
  PS-Simulink Converter/LConn1 -- theta2Rotation/RConn2
